simulink model "savareseC2"  (R2023a)
settings: Solver=FixedStepDiscrete  StartTime=0.0  StopTime=200  FixedStep=Ts  MaxStep=Ts  RelTol=1e-3
model workspace (MAT data in the model file):
  Ts = 0.002
  acoeff = 0.95
  amax = 0.1
  jcoeff = 0.1
  jmax = 1
  pf = 160
  reference_command = [0 0.002 0.004 0.006 0.008 0.01 0.012 0.014 0.016 0.018 0.02 0.022 ... (200002 elements, 100001x2)]
  v = 50
  vmax = 1.5
undefined symbols (not defined in the file or in its folder): DiscIntNeverNeededParam
(part 2 of 2)

== matlab function savareseC2/MATLAB Function2 ==
  data: param input; vout output; ds_in input
function vout = C2_dec_ramp(param,ds_in)

%% Dati

Ts = param(1);
vmax = param(2);

acoeff = param(5);
jcoeff = param(6);

amax = param(3)*acoeff;
jmax = param(4)*jcoeff;

s_switch = amax^3/(6*jmax^2);

delta_ds = amax^3/(24*jmax^2);

ds = abs(ds_in);
% valore assoluto perché il segno della traiettoria viene gestito dalla
% cascata di blocchi min e max

%% Calcolo traiettoria

v_lineare = Ts*sqrt(2*amax*abs(ds - delta_ds));
v_quad = Ts*nthroot(0.5*jmax*(3*ds).^2,3);

if ds < s_switch
    vout = v_quad;
else
    vout = v_lineare;
end

vout = sign(ds_in)*min(ds,vout);
% questa ultima riga è del tutto equivalente alla cascata di min e max

end
